simulink model "untitled"  (R2020a)
settings: Solver=VariableStepAuto  StartTime=0.0  StopTime=7  RelTol=1e-3
libraries: powerlib x9
settings Model: Creator=janke  LastModifiedBy=janke

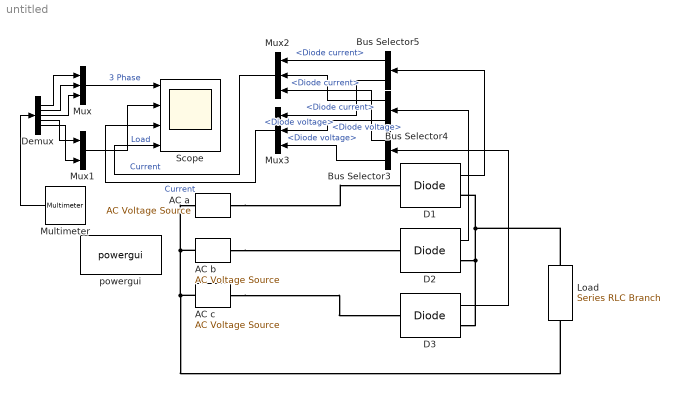
== system untitled ==
  AC a : powerlib/Electrical Sources/AC Voltage Source  Amplitude=5  Phase=0  Frequency=1  SampleTime=0  Measurements=Voltage  BusType=swing  Pref=10e3  Qref=0  Qmin=-inf  Qmax=+inf
  AC b : powerlib/Electrical Sources/AC Voltage Source  Amplitude=5  Phase=120  Frequency=1  SampleTime=0  Measurements=Voltage  BusType=swing  Pref=10e3  Qref=0  Qmin=-inf  Qmax=+inf
  AC c : powerlib/Electrical Sources/AC Voltage Source  Amplitude=5  Phase=240  Frequency=1  SampleTime=0  Measurements=Voltage  BusType=swing  Pref=10e3  Qref=0  Qmin=-inf  Qmax=+inf
  Bus Selector3 : BusSelector  OutputSignals=Diode current,Diode voltage
  Bus Selector4 : BusSelector  OutputSignals=Diode current,Diode voltage
  Bus Selector5 : BusSelector  OutputSignals=Diode current,Diode voltage
  D1 : powerlib/Power Electronics/Diode  Ron=0.001  Lon=0  Vf=0.8  IC=0  UseSnubber=0  Rs=500  Cs=250e-9  Measurements=on
  D2 : powerlib/Power Electronics/Diode  Ron=0.001  Lon=0  Vf=0.8  IC=0  UseSnubber=0  Rs=500  Cs=250e-9  Measurements=on
  D3 : powerlib/Power Electronics/Diode  Ron=0.001  Lon=0  Vf=0.8  IC=0  UseSnubber=0  Rs=500  Cs=250e-9  Measurements=on
  Demux : Demux  Outputs=5
  Load : powerlib/Elements/Series RLC Branch  LConnTagsString=__new0  RConnTagsString=__new0  BranchType=RL  Resistance=1.5  Inductance=.03  SetiL0=off  InitialCurrent=0  Capacitance=.005  Setx0=off  InitialVoltage=0  Measurements=Branch voltage and current
  Multimeter : powerlib/Measurements/Multimeter  PhasorSimulation=off  OutputType=Complex  sel=[4 3 2 1 5]  L=5  Gain=[1 1 1 1 1]  yselected={'Usrc: AC a','Usrc: AC b','Usrc: AC c','Ub: Load','Ib: Load'};  PSBOutputType=1  PSBequivalent=0  AxesSetting=[0,0.1,-100,100]  Display=0  SavedBlockNames=-11
  Mux : Mux  Inputs=3
  Mux1 : Mux  Inputs=2
  Mux2 : Mux  Inputs=3
  Mux3 : Mux  Inputs=3
  Scope : Scope  NumInputPorts=4
  powergui : powerlib/powergui  Priority=1  SimulationMode=Continuous  SampleTime=50e-6  frequency=60  Iterations=50  frequencyindice=0  Pbase=100e6  ErrMax=1e-4  UnitsV=kV  UnitsW=MW  buscounter=0  FunctionMessages=off  echomessages=off  EnableUseOfTLC=off  CurrentSourceSwitches=off  DisableSnubberDevices=off  DisableRonSwitches=off  DisableVfSwitches=off  DisplayEquations=off  AutomaticDiscreteSolvers=off  SolverType=Tustin/Backward Euler (TBE)  Interpol=off  ExternalGateDelay=off  methode=off  Ts=100  x0status=blocks  SPID=on  SwTol=0  HookPort=off  NonlinearTolerance=1e-4  nMaxIteration=100  ContinueOnMaxIteration=off  RestoreLinks=warning  ResistiveCurrentMeasurement=off  Frange=[0:2:500]  Ylog=off  Xlog=on  ShowGrid=off  save=off  variable=ZData  structure=0  ZoomFFT=off  StartTime=0.0  cycles=1  DisplayStyle=1  fundamental=60  FreqAxis=off  MaxFrequency=1000  frequencyindicesteady=1  RmsSteady=1  display=off
  wires:
  Multimeter/1 -> Demux/1
  Demux/1 -> Mux/1
  Demux/2 -> Mux/2
  Demux/3 -> Mux/3
  Mux/1 -> Scope/1  "3 Phase"
  Demux/4 -> Mux1/1
  Demux/5 -> Mux1/2
  Mux1/1 -> Scope/2  "Load"
  Bus Selector5/1 -> Mux2/1  "<Diode current>"
  Mux2/1 -> Scope/4  "Current"
  D1/1 -> Bus Selector5/1
  D2/1 -> Bus Selector4/1
  D3/1 -> Bus Selector3/1
  Bus Selector4/1 -> Mux2/2  "<Diode current>"
  Bus Selector3/1 -> Mux2/3  "<Diode current>"
  Bus Selector3/2 -> Mux3/3  "<Diode voltage>"
  Bus Selector4/2 -> Mux3/2  "<Diode voltage>"
  Bus Selector5/2 -> Mux3/1  "<Diode voltage>"
  Mux3/1 -> Scope/3  "Current"
  connections:
  AC b/LConn1 -- AC c/LConn1 -- Load/RConn1 -- AC a/LConn1
  D2/RConn1 -- D3/RConn1 -- Load/LConn1 -- D1/RConn1
  AC a/RConn1 -- D1/LConn1
  AC b/RConn1 -- D2/LConn1
  AC c/RConn1 -- D3/LConn1
